simulink model "MDCC"  (R2021b)
settings: Solver=FixedStepDiscrete  StartTime=0.0  StopTime=10.0  FixedStep=0.0001  RelTol=1e-3
model workspace (MATLAB code in the model file):
  | cmdLim = Simulink.Parameter;
  | cmdLim.Value = 15;
  | cmdLim.Description = 'Limit for controlling the maximum surface command angle.';
  | cmdLim.Min = 0;
  | cmdLim.Max = 90;
  | cmdLim.DocUnits = 'deg';
  | 
  | dispGain = Simulink.Parameter;
  | dispGain.Value = 0.75;
  | dispGain.Description = 'Gain applied to the displacement error.';
  | dispGain.Min = 0;
  | dispGain.Max = [];
  | dispGain.DocUnits = 'deg/sec/deg';
  | 
  | dispLim = Simulink.Parameter;
  | dispLim.Value = 30;
  | dispLim.Description = 'Limit for controlling the maximum commanded angle.';
  | dispLim.Min = 0;
  | dispLim.Max = 180;
  | dispLim.DocUnits = 'deg';
  | 
  | intGain = Simulink.Parameter;
  | intGain.Value = 0.5;
  | intGain.Description = 'Gain applied to the integral error.';
  | intGain.Min = 0;
  | intGain.Max = [];
  | intGain.DocUnits = 'deg/sec/deg/sec';
  | 
  | intLim = Simulink.Parameter;
  | intLim.Value = 5;
  | intLim.Description = 'Limit for controlling the maximum commanded angle.';
  | intLim.Min = 0;
  | intLim.Max = 90;
  | intLim.DocUnits = 'deg';
  | 
  | rateGain = Simulink.Parameter;
  | rateGain.Value = 2;
  | rateGain.Description = 'Gain applied to the rate error.';
  | rateGain.Min = 0;
  | rateGain.Max = [];
  | rateGain.DocUnits = 'deg/deg/sec';
  | 
  | rateLim = Simulink.Parameter;
  | rateLim.Value = 6;
  | rateLim.Description = 'Limit for controlling the maximum commanded angle.';
  | rateLim.Min = 0;
  | rateLim.Max = 180;
  | rateLim.DocUnits = 'deg/sec';
  | 
  | hdgGain = Simulink.Parameter;
  | hdgGain.Value = 0.015;
values from neighbouring files (symbols this model uses):
  KfDeadCompen_SetDeltaTime_us = myPackage.Parameter    [DeadCompen.m]
  Ts = 5E-6    (= 5e-06)    [iPMSM_data.m]
  VbDeadComp_SwtUseIsttrDes_flg = myPackage.Parameter    [DeadCompen.m]
  VfDeadCompen_ISttrDdeThdSwt_A = myPackage.Parameter    [DeadCompen.m]
  VfDeadCompen_ISttrIgbtThdSwt_A = myPackage.Parameter    [DeadCompen.m]
  VfDeadCompen_rDdeISttrHi_R = myPackage.Parameter    [DeadCompen.m]
  VfDeadCompen_rDdeISttrLo_R = myPackage.Parameter    [DeadCompen.m]
  VfDeadCompen_rIgbtISttrHi_R = myPackage.Parameter    [DeadCompen.m]
  VfDeadCompen_rIgbtISttrLo_R = myPackage.Parameter    [DeadCompen.m]
  VfDeadCompen_uDdeISttrHi_V = myPackage.Parameter    [DeadCompen.m]
  VfDeadCompen_uDdeISttrLo_V = myPackage.Parameter    [DeadCompen.m]
  VfDeadCompen_uIgbtISttrHi_V = myPackage.Parameter    [DeadCompen.m]
  VfDeadCompen_uIgbtISttrLo_V = myPackage.Parameter    [DeadCompen.m]
undefined symbols (not defined in the file or in its folder): CosTable12bit_Y, GLBCal_GLBCal_Kf_DCLinkOverVolErrThd_V, GLBCal_GLBCal_Kf_DCLinkUnderVolErrThd_V, GLBCal_GLBCal_Kf_EquiLd_NULL, GLBCal_GLBCal_Kf_EquiLq_NULL, GLBCal_GLBCal_Kf_MotorRatedSpeed_rpm, GLBCal_GLBCal_Kf_MotorSpeedHysteresis_Coef, GLBCal_Ke_MotorPolePairsNum_NULL, IoHwAbOpArg_PwmDutyCyclePhU_NULL, IoHwAbOpArg_PwmDutyCyclePhV_NULL, IoHwAbOpArg_PwmDutyCyclePhW_NULL, IoHwAbOpArg_PwmOutputEn, KbMDCC_DeadTimeCompEn_flg, KbMDCC_MCF_flgHarmInIsdqTab11ZR_flg, KbMDCC_MCF_flgHarmInIsdqTab13ZR_flg, KbMDCC_MCF_flgHarmInIsdqTab5ZR_flg, KbMDCC_MCF_flgHarmInIsdqTab7ZR_flg, KbMDCC_MCF_flgHarmInject_flg, KbMDCC_SetEAngleEn_flg, KbMDCC_UdUqFwOmit_flg, KfDeadCompen_CpPeriodTimesT_NULL, KfMDCC_ActiveDischargeIdCurVal_A, KfMDCC_ActiveDischargeIqCurVal_A, KfMDCC_DCLinkVolRate_coef, KfMDCC_DebugEAngleInit_rad, KfMDCC_DebugUalphaVolCmd_V, KfMDCC_DebugUbetaVolCmd_V, KfMDCC_DebugUdCmd_V, KfMDCC_DebugUqCmd_V, KfMDCC_DebugUsCmd_V, KfMDCC_DebugUsRate_V, KfMDCC_IMCResp_NULL, KfMDCC_IMCStab_NULL, KfMDCC_InvParkCpPeriodTimesT_NULL, KfMDCC_MCF_CircAge_NULL, KfMDCC_MCF_flgUse11Harm_flg, KfMDCC_MCF_flgUse13Harm_flg, KfMDCC_MCF_flgUse5Harm_flg, KfMDCC_MCF_flgUse7Harm_flg, KfMDCC_MCF_Harm1113FLParamSpeedThrd_rads, KfMDCC_MCF_Harm57FLParamSpeedThrd_rads, KfMDCC_MCF_HarmcofFltN_NULL, KfMDCC_MCF_HarmCpnAg_NULL, KfMDCC_MCF_HarmfLParaHigh_coef, KfMDCC_MCF_HarmfLParaLow_coef, KfMDCC_MCF_HarmIn1113ZRY_Trq_Nm, KfMDCC_MCF_HarmIn11_SpdLimHigh_rads, KfMDCC_MCF_HarmIn11_SpdLimLow_rads, KfMDCC_MCF_HarmIn11ZRY_Isd_A, KfMDCC_MCF_HarmIn11ZRY_Isq_A, KfMDCC_MCF_HarmIn13_SpdLimHigh_rads, KfMDCC_MCF_HarmIn13_SpdLimLow_rads, KfMDCC_MCF_HarmIn13ZRY_Isd_A, KfMDCC_MCF_HarmIn13ZRY_Isq_A, KfMDCC_MCF_HarmIn57ZRY_Trq_Nm, KfMDCC_MCF_HarmIn5_SpdLimHigh_rads, KfMDCC_MCF_HarmIn5_SpdLimLow_rads, KfMDCC_MCF_HarmIn5ZRY_Isd_A, KfMDCC_MCF_HarmIn5ZRY_Isq_A, KfMDCC_MCF_HarmIn7_SpdLimHigh_rads ... (+47)
libraries: simulink x40, PMSM_Library x3, mcbcontrolslib x1
(part 8 of 8)

== matlab function MDCC/DoCurCtr_sys/MDCC/UdUqCalc_Sys/UdUqCalc/IsDQCtl_m ==
  data: Decoup_coef input; PIReset input; TQC_UsdPI output; TQC_IsdDes input; TQC_IsqDes input; ISM_Isd input; ISM_Isq input; TQC_omSttr input; TQC_dtIsctl_Cc input; TQC_kidq input; TQC_kpd input; TQC_UsqPI output; TQC_kpq input; TQC_Rv input; TQC_UsqFluxExc input; TQC_uDaMax_Cc input; TQC_uQaMax_Cc input; facIntglDa_Dbg output; facIntglQa_Dbg output; facIntglDaQa_Dbg output; uDaUnlim_Dbg output; uQaUnlim_Dbg output; iDaDes_Dbg output; iQaDes_Dbg output
function [TQC_UsdPI,TQC_UsqPI,facIntglDa_Dbg,facIntglQa_Dbg,facIntglDaQa_Dbg,uDaUnlim_Dbg,uQaUnlim_Dbg,iDaDes_Dbg,iQaDes_Dbg] =fcn(Decoup_coef,PIReset,TQC_IsdDes,TQC_IsqDes,ISM_Isd,ISM_Isq,TQC_omSttr,TQC_dtIsctl_Cc,TQC_kidq,TQC_kpd,TQC_kpq,TQC_Rv,TQC_UsqFluxExc,TQC_uDaMax_Cc,TQC_uQaMax_Cc)

    persistent iDaDes iQaDes
    persistent iDaErrTust iQaErrTust
    persistent omSttr agDelta
    persistent facIntglDaQa facIntglDa facIntglQa
    persistent ydAdd yqAdd ydInt yqInt yPd yPq yRvd yRvq ydPFF yqPFF
    persistent uDaUnlim uQaUnlim 
    persistent uDaPI uQaPI
 if isempty(ydInt)
    ydInt = single(0);
    yqInt = single(0);
 end
    
 if(PIReset == 0)
    % new ramp calculation
		% correct calc
 
    iDaDes = TQC_IsdDes;
	iQaDes = TQC_IsqDes;
	

	iDaErrTust = (iDaDes - ISM_Isd)/2;
	iQaErrTust = (iQaDes - ISM_Isq)/2;
	
	omSttr = TQC_omSttr;
	agDelta = TQC_dtIsctl_Cc*omSttr*Decoup_coef;
	

	facIntglDaQa 	= TQC_kidq*TQC_dtIsctl_Cc;
	facIntglDa  	= TQC_kpd*agDelta;
	facIntglQa  	= TQC_kpq*agDelta;

	ydAdd	= facIntglDaQa*iDaErrTust - facIntglQa*iQaErrTust;
	yqAdd 	= facIntglDaQa*iQaErrTust + facIntglDa*iDaErrTust;

	ydInt   = ydInt + ydAdd;				
	yqInt   = yqInt + yqAdd;				
	
	yPd     = TQC_kpd*iDaErrTust*2;
	yPq     = TQC_kpq*iQaErrTust*2;
	yRvd    = TQC_Rv*ISM_Isd;
	yRvq    = TQC_Rv*ISM_Isq;
	
    ydPFF = yPd - yRvd;
	yqPFF = yPq - yRvq + TQC_UsqFluxExc;

	% calulation of feed forward voltage
% 	uR 			= TQC_RSttrFdFwd_Cc*iDaDesIntrpn;
% 	rIndu 		= omSttr*TQC_LQaFdFwd_Cc;
% 	uL 			= rIndu*iQaDesIntrpn;
% 	uDaFdFwd	= uR - uL;
% 	
% 	uR 			= TQC_RSttrFdFwd_Cc*iQaDesIntrpn;
% 	rIndu 		= omSttr*TQC_LDaFdFwd_Cc;
% 	uL 			= rIndu*iDaDesIntrpn;
% 	uQaFdFwd 	= uR + uL;
	
% 	if(TQC_bUseUFwdLimn_Cc)
%         % add uFdFwd before limitation
% 		ydPFF = ydPFF + uDaFdFwd;
% 		yqPFF = yqPFF + uQaFdFwd;
% 	end
	
	uDaUnlim = ydInt + ydPFF;		 
	uQaUnlim = yqInt + yqPFF;		
	
	
    if(uDaUnlim > TQC_uDaMax_Cc)
		uDaPI 		= TQC_uDaMax_Cc;
		ydInt 		= uDaPI - ydPFF;	
    else
        if(uDaUnlim < -TQC_uDaMax_Cc)
            uDaPI 	= -TQC_uDaMax_Cc;
			ydInt 	= uDaPI - ydPFF;	
        else	
			uDaPI 	= uDaUnlim;
			ydInt 	= ydInt + ydAdd;			
        end
    end


    if(uQaUnlim > TQC_uQaMax_Cc)
		uQaPI		= TQC_uQaMax_Cc;
		yqInt 		= uQaPI - yqPFF;	
    else
        if(uQaUnlim < -TQC_uQaMax_Cc)
			uQaPI	= -TQC_uQaMax_Cc;
			yqInt	= uQaPI - yqPFF;	
        else	
			uQaPI	= uQaUnlim;
			yqInt	= yqInt + yqAdd;			
        end
    end
	
%     if(TQC_bUseUFwdLimn_Cc == 0)
%         % add uFdFwd after limitation
% 		uDaPI = uDaPI + uDaFdFwd;
% 		uQaPI = uQaPI + uQaFdFwd;
%     end

	TQC_UsdPI = uDaPI;
	TQC_UsqPI = uQaPI;
	
    % 	Debug 
 	facIntglDa_Dbg      = facIntglDa;
 	facIntglQa_Dbg      = facIntglQa;
 	facIntglDaQa_Dbg    = facIntglDaQa;
 	uDaUnlim_Dbg        = uDaUnlim;
 	uQaUnlim_Dbg        = uQaUnlim;
 	iDaDes_Dbg          = iDaDes;
 	iQaDes_Dbg          = iQaDes;
% 	uDaFdFwd_Dbg        = uDaFdFwd;
% 	uQaFdFwd_Dbg        = uQaFdFwd;

else 
	ydInt	= single(0);
	yqInt	= single(0);
	TQC_UsdPI = single(0);
	TQC_UsqPI = single(0);
    facIntglDa_Dbg = single(0);
    facIntglQa_Dbg = single(0);
    facIntglDaQa_Dbg = single(0);
    uDaUnlim_Dbg = single(0);
    uQaUnlim_Dbg = single(0);
    iDaDes_Dbg = single(0);
    iQaDes_Dbg = single(0); 
 end

== stateflow chart MDCC/DoCurCtr_sys/MDCC/IrmsCalc_Sys/Chart ==
  (default) -> (junction 1)
  (junction 1) -> (junction 5) : {First}
  (junction 5) -> (junction 6) : {Second}
  (junction 6) -> (junction 8) : {Thrid}
  (junction 8) -> (junction 10)
  events: First output FUNCTION_CALL_EVENT; Second output FUNCTION_CALL_EVENT; Thrid output FUNCTION_CALL_EVENT

== stateflow chart MDCC/DoCurCtr_sys/MDCC/MDCC_State ==
  note: Do not put any code along
      | the transitions that run
      | down the right side!
  (default) -> (junction 431)
  (junction 431) -> (junction 428) [order 1] : [VuMDSM_MCUStatus_NULL == MDSM_MCUStatus.MDSM_ActiveDischarge ]
      | {
      | VbMDCC_PIRstEn_flg = false;
      | MDCC_PWMEn = true;
      | }
  (junction 431) -> (junction 280) [order 2]
  (junction 428) -> (junction 384) : {
      |       ResEAngle_Calc;
      | 	VbMDCC_UdUqCalc1Enb_flg = true;
      |       VbMDCC_UdUqCalc2Enb_flg = false;
      |       VbMDCC_SelfHeatingEn_flg = false;
      | 	UdUqCalc;
      |
      | 	//MDCC_Inverse_Park_rotation_coef_cp_Call;
      | 	//MDCC_Inverse_Park_Transform_Call;
      | 	//MDCC_Inverse_Clark_Transform_Call;
      | 	MDCC_MDSA_Call;
      |      // VeMDSM_PWMOutMode_enum = MDCC_PWMOUTMODE.NORMAL;
      | }
  (junction 382) -> (junction 384) : {
      |       VbMDCC_UdUqCalc1Enb_flg = true;
      |       VbMDCC_UdUqCalc2Enb_flg = false;
      |       VbMDCC_SelfHeatingEn_flg = false;
      |
      |       VfMDSA_PwmDutyCyclePhaseU_NULL = 0.5f;
      | 	VfMDSA_PwmDutyCyclePhaseV_NULL = 0.5f;
      | 	VfMDSA_PwmDutyCyclePhaseW_NULL = 0.5f;
      | }
  (junction 272) -> (junction 382) [order 1] : [MDSP_VbMDSP_HardwareASC_flg == true]
  (junction 384) -> (junction 282)
  (junction 280) -> (junction 281) [order 1] : [VbMDFM_EmergeStopEnb_flg == true]
      | {
      | VbMDCC_PIRstEn_flg = true;
      | MDCC_PWMEn = false;
      | VbMDCC_SelfHeatingEn_flg = false;
      | UdUqCalc;
      | }
  (junction 281) -> (junction 272) [order 1] : [VbMDCC_MotorASCEn_flg == true]//VfMDSP_MotorAveAbsSpeed_rpm > KfMDSP_MotorRatedSpeed_rpm]//||VbMDFM_EmergencyShutoff_flg==true]
  (junction 272) -> (junction 282) [order 2] : {
      | 	VbMDCC_UdUqCalc1Enb_flg = true;
      |       VbMDCC_UdUqCalc2Enb_flg = false;
      |       VbMDCC_SelfHeatingEn_flg = false;
      |
      |       //VeMDSM_PWMOutMode_enum 	= MDCC_PWMOUTMODE.TOP_OFF_BOTTOM_OFF;
      |
      | 	//VbMDCC_UdUqCalc1Enb_flg = false;
      |       //VbMDCC_UdUqCalc2Enb_flg = false;
      |       //UdUqCalc;
      | 	//VfMDCC_UdVal_V = 0.0f;
      | 	//VfMDCC_UqVal_V = 0.0f;
      | 	//VfMDCC_UalphaVol_V = 0.0f;
      | 	//VfMDCC_UbetaVol_V = 0.0f;
      |
      | 	VfMDSA_PwmDutyCyclePhaseU_NULL = 0.5f;
      | 	VfMDSA_PwmDutyCyclePhaseV_NULL = 0.5f;
      | 	VfMDSA_PwmDutyCyclePhaseW_NULL = 0.5f;
      |
      |      //MDCC_ASC_Call;
      |      VbMDCC_ASCEnable_flg = true;
      | }
  (junction 280) -> (junction 268) [order 2] : { VbMDCC_ASCEnable_flg = false}
  (junction 281) -> (junction 413) [order 2]
  (junction 282) -> (junction 279)
  (junction 413) -> (junction 415) [order 1] : [MDSP_VbMDSP_HardwareFW_flg == true]
  (junction 413) -> (junction 411) [order 2] : {MDCC_FW_Call}
  (junction 415) -> (junction 417)
  (junction 417) -> (junction 411)
  (junction 411) -> (junction 283) : //[VeMDSM_PWMOutMode_enum != MDCC_PWMOUTMODE.TOP_OFF_BOTTOM_OFF]
  (junction 283) -> (junction 380) : {
      |       VbMDCC_UdUqCalc1Enb_flg = true;
      |       VbMDCC_UdUqCalc2Enb_flg = false;
      |       VbMDCC_SelfHeatingEn_flg = false;
      |      VbMDCC_ASCEnable_flg = false;
      | 	//UdUqCalc;
      | 	//MDCC_Inverse_Park_rotation_coef_cp_Call;
      | 	//MDCC_Inverse_Park_Transform_Call;
      | 	//MDCC_Inverse_Clark_Transform_Call;
      | 	//MDCC_MDSA_Call;
      |
      |       VfMDSA_PwmDutyCyclePhaseU_NULL = 0.5f;
      | 	VfMDSA_PwmDutyCyclePhaseV_NULL = 0.5f;
      | 	VfMDSA_PwmDutyCyclePhaseW_NULL = 0.5f;
      |
      |       //MDCC_FW_Call;
      |
      |       //VeMDSM_PWMOutMode_enum = MDCC_PWMOUTMODE.NORMAL;
      | }
  (junction 380) -> (junction 279)
  (junction 279) -> (junction 271)
  (junction 268) -> (junction 269) [order 1] : [(VuMDSM_MCUStatus_NULL == MDSM_MCUStatus.MDSM_TorqueControl) || (VuMDSM_MCUStatus_NULL == MDSM_MCUStatus.MDSM_SpeedControl)]
      | {
      | VbMDCC_PIRstEn_flg = false;
      | MDCC_PWMEn = true;
      | }
  (junction 268) -> (junction 273) [order 2]
  (junction 269) -> (junction 270) : {
      |       ResEAngle_Calc;
      | 	VbMDCC_UdUqCalc1Enb_flg = true;
      |       VbMDCC_UdUqCalc2Enb_flg = false;
      |       VbMDCC_SelfHeatingEn_flg = false;
      | 	UdUqCalc;
      |
      | 	//MDCC_Inverse_Park_rotation_coef_cp_Call;
      | 	//MDCC_Inverse_Park_Transform_Call;
      | 	//MDCC_Inverse_Clark_Transform_Call;
      | 	MDCC_MDSA_Call;
      |      // VeMDSM_PWMOutMode_enum = MDCC_PWMOUTMODE.NORMAL;
      | }
  (junction 270) -> (junction 271)
  (junction 271) -> (junction 300)
  (junction 273) -> (junction 274) [order 1] : [(VuMDSM_MCUStatus_NULL == MDSM_MCUStatus.MDSM_DebugHandle)]
      | {
      | VbMDCC_PIRstEn_flg = false;
      | MDCC_PWMEn = true;
      | }
  (junction 273) -> (junction 398) [order 2]
  (junction 274) -> (junction 275)
  (junction 275) -> (junction 276) [order 1] : [VeMDST_MDSMDebugMode_NULL == MDSM_DEBUG.MDSM_IdIqMODE]
  (junction 275) -> (junction 314) [order 2]
  (junction 276) -> (junction 277) : {
      |       ResEAngle_Calc;
      | 	VbMDCC_UdUqCalc1Enb_flg = true;
      |       VbMDCC_UdUqCalc2Enb_flg = false;
      |       VbMDCC_SelfHeatingEn_flg = false;
      | 	UdUqCalc;
      | 	//MDCC_Inverse_Park_rotation_coef_cp_Call;
      | 	//MDCC_Inverse_Park_Transform_Call;
      | 	//MDCC_Inverse_Clark_Transform_Call;
      | 	MDCC_MDSA_Call;
      |       //VeMDSM_PWMOutMode_enum = MDCC_PWMOUTMODE.NORMAL;
      | }
  (junction 277) -> (junction 300)
  (junction 300) -> (junction 308)
  (junction 314) -> (junction 309) [order 1] : [VeMDST_MDSMDebugMode_NULL == MDSM_DEBUG.MDSM_UdUqMODE]
  (junction 314) -> (junction 310) [order 2]
  (junction 309) -> (junction 293) : {
      |       ResEAngle_Calc;
      | 	VbMDCC_UdUqCalc1Enb_flg = false;
      |       VbMDCC_UdUqCalc2Enb_flg = true;
      |       VbMDCC_SelfHeatingEn_flg = false;
      |       UdUqCalc;
      | 	//MDCC_Inverse_Park_rotation_coef_cp_Call;
      | 	//MDCC_Inverse_Park_Transform_Call;
      | 	//MDCC_Inverse_Clark_Transform_Call;
      | 	MDCC_MDSA_Call;
      | 	//VeMDSM_PWMOutMode_enum = MDCC_PWMOUTMODE.NORMAL;
      | }
  (junction 293) -> (junction 308)
  (junction 308) -> (junction 301)
  (junction 310) -> (junction 286) [order 1] : [VeMDST_MDSMDebugMode_NULL == MDSM_DEBUG.MDSM_UaUbMODE]
  (junction 310) -> (junction 289) [order 2]
  (junction 286) -> (junction 291) : {
      | 	MDCC_DebugUaUb_Call;
      | 	MDCC_MDSA_Call;
      | 	//VeMDSM_PWMOutMode_enum = MDCC_PWMOUTMODE.NORMAL;
      | }
  (junction 291) -> (junction 301)
  (junction 301) -> (junction 312)
  (junction 289) -> (junction 311) [order 1] : [VeMDST_MDSMDebugMode_NULL == MDSM_DEBUG.MDSM_UsMODE]
  (junction 289) -> (junction 303) [order 2]
  (junction 311) -> (junction 302) : {
      | 	MDCC_DebugUs_Call;
      | 	MDCC_MDSA_Call;
      | 	VeMDSM_PWMOutMode_enum = MDCC_PWMOUTMODE.NORMAL;
      | }
  (junction 302) -> (junction 312)
  (junction 312) -> (junction 290)
  (junction 303) -> (junction 292) : [VeMDST_MDSMDebugMode_NULL == MDSM_DEBUG.MDSM_IfMODE]
  (junction 292) -> (junction 304) : {
      |      AutoEAngle_Calc;
      |      VbMDCC_UdUqCalc1Enb_flg = true;
      |       VbMDCC_UdUqCalc2Enb_flg = false;
      |       VbMDCC_SelfHeatingEn_flg = false;
      |
      | 	UdUqCalc;
      | 	//MDCC_Inverse_Park_rotation_coef_cp_Call;
      | 	//MDCC_Inverse_Park_Transform_Call;
      | 	//MDCC_Inverse_Clark_Transform_Call;
      | 	MDCC_MDSA_Call;
      |       //VeMDSM_PWMOutMode_enum = MDCC_PWMOUTMODE.NORMAL;
      | }
  (junction 398) -> (junction 400) [order 1] : [VbMDSP_McuFSelfheatingMode_flg == true || VbMDCC_PreSelfHeatingStop_flg == false ]{MDCC_PWMEn = true;}
  (junction 398) -> (junction 305) [order 2]
  (junction 400) -> (junction 402) : {
      | ResEAngle_Calc;
      | VbMDCC_UdUqCalc1Enb_flg = false;
      | VbMDCC_UdUqCalc2Enb_flg = false;
      | VbMDCC_SelfHeatingEn_flg = true;
      | UdUqCalc;
      | MDCC_MDSA_Call;
      | }
  (junction 304) -> (junction 290)
  (junction 290) -> (junction 288)
  (junction 305) -> (junction 313) [commented out] : [VeMDPM_MCUStatus_NULL == MDPM_MCUStatus.MDPM_AFTERRUN2 ]
  (junction 305) -> (junction 306) : {	//VeMDSM_PWMOutMode_enum 	= MDCC_PWMOUTMODE.TOP_OFF_BOTTOM_OFF;
      |
      | 	//VbMDCC_UdUqCalc1Enb_flg = false;
      |       //VbMDCC_UdUqCalc2Enb_flg = false;
      |       //UdUqCalc;
      | 	//VfMDCC_UdVal_V = 0.0f;
      | 	//VfMDCC_UqVal_V = 0.0f;
      | 	//VfMDCC_UalphaVol_V = 0.0f;
      | 	//VfMDCC_UbetaVol_V = 0.0f;
      |
      |       MDCC_PWMEn = false;
      |       MDCC_FW_Call;
      | 	VfMDSA_PwmDutyCyclePhaseU_NULL = 0.5f;
      | 	VfMDSA_PwmDutyCyclePhaseV_NULL = 0.5f;
      | 	VfMDSA_PwmDutyCyclePhaseW_NULL = 0.5f;
      |       VbMDCC_PIRstEn_flg = true;
      |       VbMDCC_UdUqCalc1Enb_flg = true;
      |       VbMDCC_UdUqCalc2Enb_flg = false;
      |       VbMDCC_SelfHeatingEn_flg = false;
      |       UdUqCalc;
      |
      | }
  (junction 313) -> (junction 307) [commented out] : {
      |      // VeMDSM_PWMOutMode_enum 	= MDCC_PWMOUTMODE.NORMAL;
      | 	VfMDSA_PwmDutyCyclePhaseU_NULL = 0.5f;
      | 	VfMDSA_PwmDutyCyclePhaseV_NULL = 0.5f;
      | 	VfMDSA_PwmDutyCyclePhaseW_NULL = 0.5f;
      | }
  (junction 307) -> (junction 306)
  (junction 402) -> (junction 307)
  (junction 288) -> (junction 402)
  (junction 306) -> (junction 299)
  data: MDSP_VbMDSP_HardwareFW_flg input; MDSP_VbMDSP_HardwareASC_flg input; VuMDSM_MCUStatus_NULL input; VeMDST_MDSMDebugMode_NULL input; VeMDSM_PWMOutMode_enum output uint8; VfMDSA_PwmDutyCyclePhaseU_NULL output single; VfMDSA_PwmDutyCyclePhaseV_NULL output single; VfMDSA_PwmDutyCyclePhaseW_NULL output single; VbMDCC_UdUqCalc1Enb_flg output boolean; VbMDCC_UdUqCalc2Enb_flg output boolean; VbMDFM_EmergeStopEnb_flg input; VbMDCC_MotorASCEn_flg input; VbMDFM_EmergencyShutoff_flg input boolean [0..1]; VbMDCC_PIRstEn_flg output boolean =true; MDCC_PWMEn output boolean =false; VbMDFM_HwErrL3_flg input; VbMDCC_ASCEnable_flg output boolean =false; VbMDSP_McuFSelfheatingMode_flg input; VbMDCC_SelfHeatingEn_flg output double; VbMDCC_PreSelfHeatingStop_flg input
  events: MDCC_MDSA_Call output FUNCTION_CALL_EVENT; MDCC_DebugUaUb_Call output FUNCTION_CALL_EVENT; MDCC_DebugUs_Call output FUNCTION_CALL_EVENT; UdUqCalc output FUNCTION_CALL_EVENT; MDCC_FW_Call output FUNCTION_CALL_EVENT; AutoEAngle_Calc output FUNCTION_CALL_EVENT; ResEAngle_Calc output FUNCTION_CALL_EVENT

== matlab function MDCC/DoCurCtr_sys/MDCC/UdUqCalc_Sys/UdUqCalc/IsDQCtl_200us/IsDQCtl_m ==
  data: PIReset input; TQC_UsdPI output; TQC_IsdDes input; TQC_IsqDes input; ISM_Isd input; ISM_Isq input; TQC_omSttr input; TQC_dtIsctl_Cc input; TQC_kidq input; TQC_kpd input; TQC_UsqPI output; TQC_kpq input; TQC_Rv input; TQC_UsqFluxExc input; TQC_uDaMax_Cc input; TQC_uQaMax_Cc input; facIntglDa_Dbg output; facIntglQa_Dbg output; facIntglDaQa_Dbg output; uDaUnlim_Dbg output; uQaUnlim_Dbg output; iDaDes_Dbg output; iQaDes_Dbg output
function [TQC_UsdPI,TQC_UsqPI,facIntglDa_Dbg,facIntglQa_Dbg,facIntglDaQa_Dbg,uDaUnlim_Dbg,uQaUnlim_Dbg,iDaDes_Dbg,iQaDes_Dbg] =fcn(PIReset,TQC_IsdDes,TQC_IsqDes,ISM_Isd,ISM_Isq,TQC_omSttr,TQC_dtIsctl_Cc,TQC_kidq,TQC_kpd,TQC_kpq,TQC_Rv,TQC_UsqFluxExc,TQC_uDaMax_Cc,TQC_uQaMax_Cc)

    persistent iDaDes iQaDes
    persistent iDaErrTust iQaErrTust
    persistent omSttr agDelta
    persistent facIntglDaQa facIntglDa facIntglQa
    persistent ydAdd yqAdd ydInt yqInt yPd yPq yRvd yRvq ydPFF yqPFF
    persistent uDaUnlim uQaUnlim 
    persistent uDaPI uQaPI
 if isempty(ydInt)
    ydInt = single(0);
    yqInt = single(0);
 end
    
 if(PIReset == 0)
    % new ramp calculation
		% correct calc
 
    iDaDes = TQC_IsdDes;
	iQaDes = TQC_IsqDes;
	

	iDaErrTust = (iDaDes - ISM_Isd)/2;
	iQaErrTust = (iQaDes - ISM_Isq)/2;
	
	omSttr = TQC_omSttr;
	agDelta = TQC_dtIsctl_Cc*omSttr;
	

	facIntglDaQa 	= TQC_kidq*TQC_dtIsctl_Cc;
	facIntglDa  	= TQC_kpd*agDelta;
	facIntglQa  	= TQC_kpq*agDelta;

	ydAdd	= facIntglDaQa*iDaErrTust - facIntglQa*iQaErrTust;
	yqAdd 	= facIntglDaQa*iQaErrTust + facIntglDa*iDaErrTust;

	ydInt   = ydInt + ydAdd;				
	yqInt   = yqInt + yqAdd;				
	
	yPd     = TQC_kpd*iDaErrTust*2;
	yPq     = TQC_kpq*iQaErrTust*2;
	yRvd    = TQC_Rv*ISM_Isd;
	yRvq    = TQC_Rv*ISM_Isq;
	
    ydPFF = yPd - yRvd;
	yqPFF = yPq - yRvq + TQC_UsqFluxExc;

	% calulation of feed forward voltage
% 	uR 			= TQC_RSttrFdFwd_Cc*iDaDesIntrpn;
% 	rIndu 		= omSttr*TQC_LQaFdFwd_Cc;
% 	uL 			= rIndu*iQaDesIntrpn;
% 	uDaFdFwd	= uR - uL;
% 	
% 	uR 			= TQC_RSttrFdFwd_Cc*iQaDesIntrpn;
% 	rIndu 		= omSttr*TQC_LDaFdFwd_Cc;
% 	uL 			= rIndu*iDaDesIntrpn;
% 	uQaFdFwd 	= uR + uL;
	
% 	if(TQC_bUseUFwdLimn_Cc)
%         % add uFdFwd before limitation
% 		ydPFF = ydPFF + uDaFdFwd;
% 		yqPFF = yqPFF + uQaFdFwd;
% 	end
	
	uDaUnlim = ydInt + ydPFF;		 
	uQaUnlim = yqInt + yqPFF;		
	
	
    if(uDaUnlim > TQC_uDaMax_Cc)
		uDaPI 		= TQC_uDaMax_Cc;
		ydInt 		= uDaPI - ydPFF;	
    else
        if(uDaUnlim < -TQC_uDaMax_Cc)
            uDaPI 	= -TQC_uDaMax_Cc;
			ydInt 	= uDaPI - ydPFF;	
        else	
			uDaPI 	= uDaUnlim;
			ydInt 	= ydInt + ydAdd;			
        end
    end


    if(uQaUnlim > TQC_uQaMax_Cc)
		uQaPI		= TQC_uQaMax_Cc;
		yqInt 		= uQaPI - yqPFF;	
    else
        if(uQaUnlim < -TQC_uQaMax_Cc)
			uQaPI	= -TQC_uQaMax_Cc;
			yqInt	= uQaPI - yqPFF;	
        else	
			uQaPI	= uQaUnlim;
			yqInt	= yqInt + yqAdd;			
        end
    end
	
%     if(TQC_bUseUFwdLimn_Cc == 0)
%         % add uFdFwd after limitation
% 		uDaPI = uDaPI + uDaFdFwd;
% 		uQaPI = uQaPI + uQaFdFwd;
%     end

	TQC_UsdPI = uDaPI;
	TQC_UsqPI = uQaPI;
	
    % 	Debug 
 	facIntglDa_Dbg      = facIntglDa;
 	facIntglQa_Dbg      = facIntglQa;
 	facIntglDaQa_Dbg    = facIntglDaQa;
 	uDaUnlim_Dbg        = uDaUnlim;
 	uQaUnlim_Dbg        = uQaUnlim;
 	iDaDes_Dbg          = iDaDes;
 	iQaDes_Dbg          = iQaDes;
% 	uDaFdFwd_Dbg        = uDaFdFwd;
% 	uQaFdFwd_Dbg        = uQaFdFwd;

else 
	ydInt	= single(0);
	yqInt	= single(0);
	TQC_UsdPI = single(0);
	TQC_UsqPI = single(0);
    facIntglDa_Dbg = single(0);
    facIntglQa_Dbg = single(0);
    facIntglDaQa_Dbg = single(0);
    uDaUnlim_Dbg = single(0);
    uQaUnlim_Dbg = single(0);
    iDaDes_Dbg = single(0);
    iQaDes_Dbg = single(0); 
 end
